simulink model "tutorial09_state_space"  (R2025a)
settings: Solver=VariableStepAuto  StartTime=0.0  StopTime=10  RelTol=1e-3
settings Model: Creator=xing2  LastModifiedBy=xing2

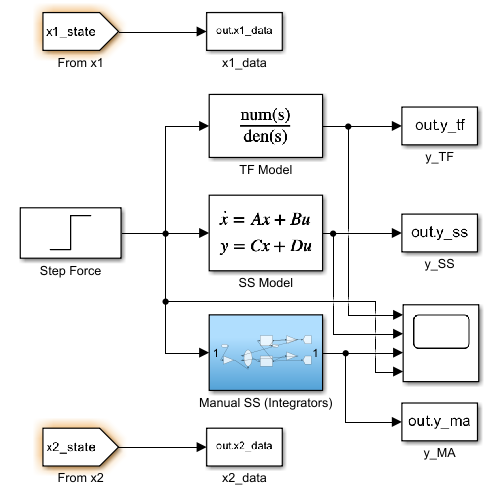
[thumbnail: Simulink's stored preview of the top-level diagram]
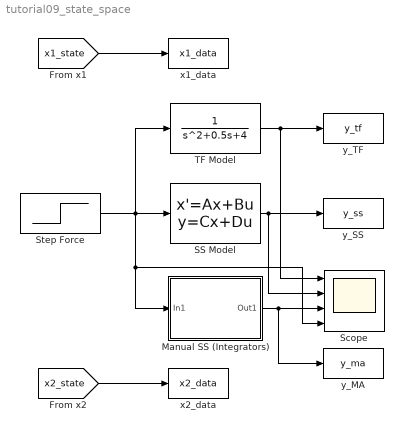
== system tutorial09_state_space ==
  Manual SS (Integrators) : Subsystem
  SS Model : StateSpace  A=[0 1;-4 -0.5]  B=[0;1]  C=[1 0]  D=0  InitialCondition=[0; 0]
  Scope : Scope  NumInputPorts=4
  Step Force : Step  SampleTime=0
  TF Model : TransferFcn  Numerator=1  Denominator=[1 0.5 4]
  x1_data : ToWorkspace  VariableName=x1_data  SaveFormat=Timeseries  SampleTime=-1
  x2_data : ToWorkspace  VariableName=x2_data  SaveFormat=Timeseries  SampleTime=-1
  y_MA : ToWorkspace  VariableName=y_ma  SaveFormat=Timeseries  SampleTime=-1
  y_SS : ToWorkspace  VariableName=y_ss  SaveFormat=Timeseries  SampleTime=-1
  y_TF : ToWorkspace  VariableName=y_tf  SaveFormat=Timeseries  SampleTime=-1
  wires:
  [x2_state] -> x2_data/1
  [x1_state] -> x1_data/1
  Step Force/1 -> Manual SS (Integrators)/1(In1), Scope/4, SS Model/1, TF Model/1
  TF Model/1 -> Scope/1, y_TF/1
  SS Model/1 -> Scope/2, y_SS/1
  Manual SS (Integrators)/1(Out1) -> Scope/3, y_MA/1

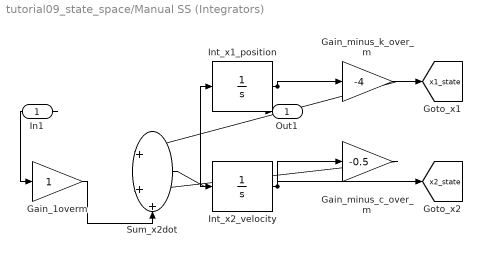
== system tutorial09_state_space/Manual SS (Integrators) ==
  In1 : Inport
  Gain_1overm : Gain
  Gain_minus_c_over_m : Gain  Gain=-0.5
  Gain_minus_k_over_m : Gain  Gain=-4
  Int_x1_position : Integrator
  Int_x2_velocity : Integrator
  Sum_x2dot : Sum  Inputs=|+++
  Out1 : Outport
  tag scope: x1_state=global, x2_state=global
  wires:
  In1/1 -> Gain_1overm/1
  Gain_1overm/1 -> Sum_x2dot/3
  Sum_x2dot/1 -> Int_x2_velocity/1
  Int_x2_velocity/1 -> Int_x1_position/1, Gain_minus_c_over_m/1, [x2_state]
  Int_x1_position/1 -> Gain_minus_k_over_m/1, [x1_state], Out1/1
  Gain_minus_k_over_m/1 -> Sum_x2dot/1
  Gain_minus_c_over_m/1 -> Sum_x2dot/2
